simulink model "trackingSim"  (R2016a)
settings: Solver=FixedStepAuto  StartTime=0.0  StopTime=T  FixedStep=dt  RelTol=1e-3
values from neighbouring files (symbols this model uses):
  a = 80*pi/180    (= 1.3962634016)    [MainCleanedUp.m]
  C = C+1    (= 1)    [dbscan.m]
  k = k + 1    (= 2)    [MainCleanedUp.m]    (also in dbscan.m)
  z0m = zeros(1,8)    [MainCleanedUp.m]
undefined symbols (not defined in the file or in its folder): Ak, Ak_1, B, B1, Bk, Bk_1, C1, Ck, Ck_1, Dk, Dk_1, F, F1, z0c
settings Model: Creator=gp1616  LastModifiedBy=gp1616

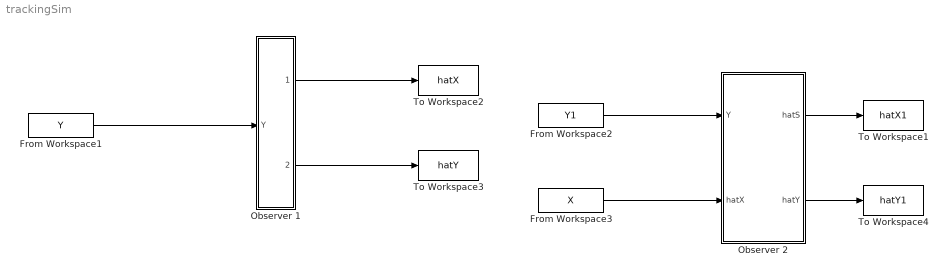
== system trackingSim ==
  From Workspace1 : FromWorkspace  VariableName=Y  SampleTime=0
  From Workspace2 : FromWorkspace  VariableName=Y1  SampleTime=0
  From Workspace3 : FromWorkspace  VariableName=X  SampleTime=0
  Observer 1 : Subsystem
  Observer 2 : Subsystem
  To Workspace1 : ToWorkspace  VariableName=hatX1  SaveFormat=Timeseries  SampleTime=-1
  To Workspace2 : ToWorkspace  VariableName=hatX  SaveFormat=Timeseries  SampleTime=-1
  To Workspace3 : ToWorkspace  VariableName=hatY  SaveFormat=Timeseries  SampleTime=-1
  To Workspace4 : ToWorkspace  VariableName=hatY1  SaveFormat=Timeseries  SampleTime=-1
  wires:
  Observer 1/1(hatX) -> To Workspace2/1
  Observer 1/2(hatY) -> To Workspace3/1
  From Workspace1/1 -> Observer 1/1("Y ")
  Observer 2/1("hatS ") -> To Workspace1/1
  Observer 2/2(hatY) -> To Workspace4/1
  From Workspace2/1 -> Observer 2/1("Y ")
  From Workspace3/1 -> Observer 2/2("hatX ")

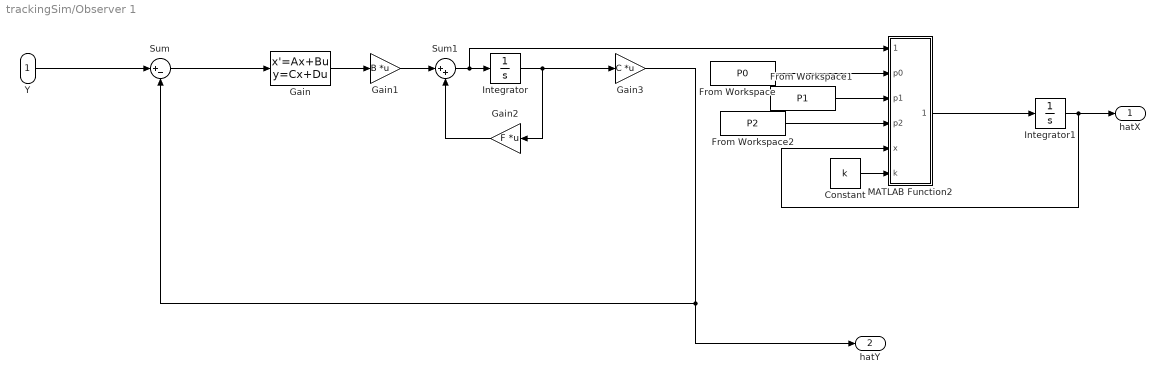
== system trackingSim/Observer 1 ==
  "Y " : Inport
  Constant : Constant  Value=k
  From Workspace : FromWorkspace  VariableName=P0  SampleTime=0
  From Workspace1 : FromWorkspace  VariableName=P1  SampleTime=0
  From Workspace2 : FromWorkspace  VariableName=P2  SampleTime=0
  Gain : StateSpace  A=Ak  B=Bk  C=Ck  D=Dk  X0=zeros(18,1)
  Gain1 : Gain  Gain=B  Multiplication=Matrix(K*u) (u vector)
  Gain2 : Gain  Gain=F  Multiplication=Matrix(K*u) (u vector)
  Gain3 : Gain  Gain=C  Multiplication=Matrix(K*u) (u vector)
  Integrator : Integrator  InitialCondition=z0c
  Integrator1 : Integrator  InitialCondition=zeros(12,1)
  MATLAB Function2 : MATLAB Function  TreatAsAtomicUnit=on
  Sum : Sum  Inputs=|+-
  Sum1 : Sum  Inputs=|++
  hatX : Outport
  hatY : Outport  Port=2
  wires:
  MATLAB Function2/1(hatx) -> Integrator1/1
  From Workspace1/1 -> MATLAB Function2/3(p1)
  From Workspace/1 -> MATLAB Function2/2(p0)
  From Workspace2/1 -> MATLAB Function2/4(p2)
  Sum1/1 -> MATLAB Function2/1(dotz), Integrator/1
  Integrator1/1 -> hatX/1, MATLAB Function2/5(x)
  Gain2/1 -> Sum1/2
  Integrator/1 -> Gain3/1, Gain2/1
  Gain3/1 -> Sum/2, hatY/1
  Sum/1 -> Gain/1
  Gain/1 -> Gain1/1
  Gain1/1 -> Sum1/1
  Constant/1 -> MATLAB Function2/6(k)
  "Y "/1 -> Sum/1

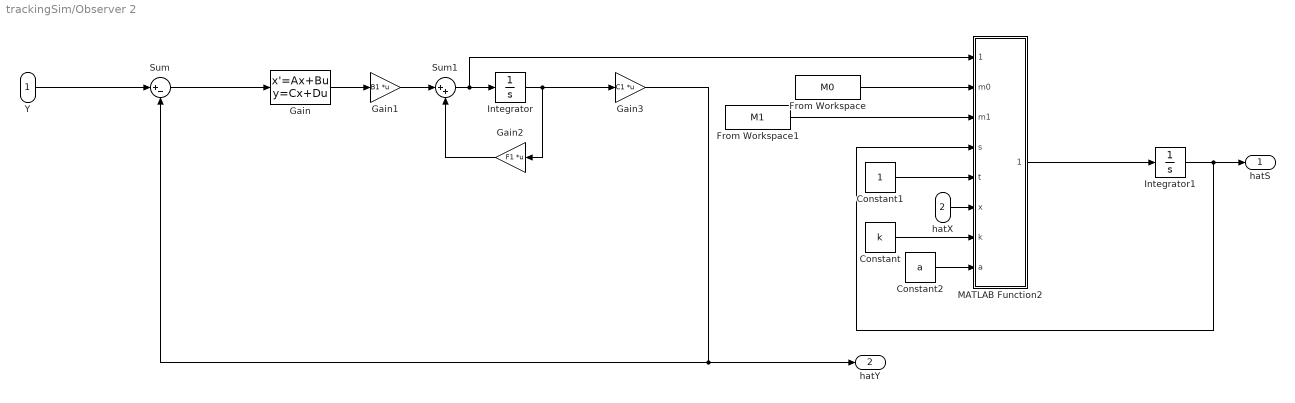
== system trackingSim/Observer 2 ==
  "Y " : Inport
  "hatX " : Inport  Port=2
  Constant : Constant  Value=k
  Constant1 : Constant
  Constant2 : Constant  Value=a
  From Workspace : FromWorkspace  VariableName=M0  SampleTime=0
  From Workspace1 : FromWorkspace  VariableName=M1  SampleTime=0
  Gain : StateSpace  A=Ak_1  B=Bk_1  C=Ck_1  D=Dk_1  X0=zeros(4,1)
  Gain1 : Gain  Gain=B1  Multiplication=Matrix(K*u) (u vector)
  Gain2 : Gain  Gain=F1  Multiplication=Matrix(K*u) (u vector)
  Gain3 : Gain  Gain=C1  Multiplication=Matrix(K*u) (u vector)
  Integrator : Integrator  InitialCondition=z0m
  Integrator1 : Integrator  InitialCondition=zeros(4,1)
  MATLAB Function2 : MATLAB Function  TreatAsAtomicUnit=on
  Sum : Sum  Inputs=|+-
  Sum1 : Sum  Inputs=|++
  "hatS " : Outport
  hatY : Outport  Port=2
  wires:
  MATLAB Function2/1(hat_s) -> Integrator1/1
  "Y "/1 -> Sum/1
  From Workspace1/1 -> MATLAB Function2/3(m1)
  From Workspace/1 -> MATLAB Function2/2(m0)
  Sum1/1 -> MATLAB Function2/1(dots), Integrator/1
  Integrator1/1 -> "hatS "/1, MATLAB Function2/4(s)
  Gain2/1 -> Sum1/2
  Integrator/1 -> Gain3/1, Gain2/1
  Gain3/1 -> hatY/1, Sum/2
  Sum/1 -> Gain/1
  Gain/1 -> Gain1/1
  Gain1/1 -> Sum1/1
  Constant/1 -> MATLAB Function2/7(k)
  Constant1/1 -> MATLAB Function2/5(t)
  Constant2/1 -> MATLAB Function2/8(a)
  "hatX "/1 -> MATLAB Function2/6(x)

== matlab function trackingSim/Observer 2/MATLAB Function2 ==
  data: dots input; m0 input; hat_s output; m1 input; s input; t input; x input; k input; a input
function hat_s = Jacobian1(dots, m0 ,m1, s, t, x, k, a)


J = Jac1(a,k,m0,m1,s,t,x);
rank(J)
hat_s = pinv(J)*dots;

end

== matlab function trackingSim/Observer 1/MATLAB Function2 ==
  data: dotz input; p0 input; hatx output; p1 input; p2 input; x input; k input
function hatx = Jacobian(dotz, p0 ,p1, p2, x, k)


J = Jac(k,p0,p1,p2,x);

%hatx = J\dotz;
if issparse(J), R = qr(J); 
else R = triu(qr(J)); end
x = R\(R'\(J'*dotz));
r = dotz - J*x;
err = R\(R'\(J'*r));
hatx = x + err;

end
